simulink model "NOLCOlab2Q2"  (R2016b)
settings: Solver=ode4  StartTime=0.0  StopTime=10.0  FixedStep=0.001  RelTol=1e-3
settings Model: Creator=akshita_jain  LastModifiedBy=akshita_jain

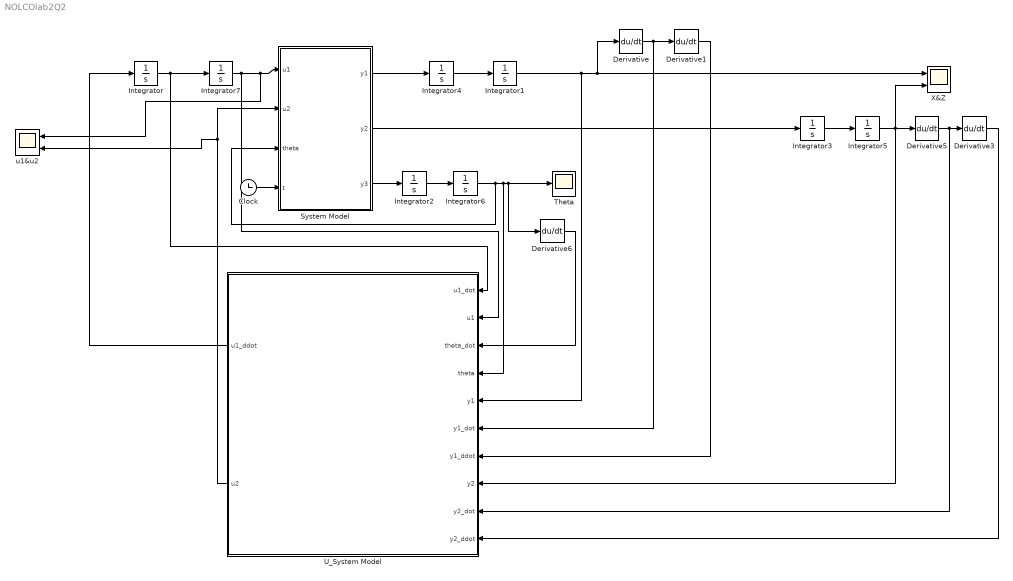
== system NOLCOlab2Q2 ==
  Clock : Clock
  Derivative{,1,3,5..6} (5 alike) : Derivative
  Integrator{,2..3,5..6} (5 alike) : Integrator
  Integrator1 : Integrator  InitialCondition=1
  Integrator4 : Integrator  InitialCondition=1
  Integrator7 : Integrator  InitialCondition=1
  System Model : MATLAB Function  TreatAsAtomicUnit=on
  Theta : Scope
  U_System Model : MATLAB Function  TreatAsAtomicUnit=on
  X&Z : Scope  NumInputPorts=2
  u1&u2 : Scope  NumInputPorts=2
  wires:
  System Model/2(y2) -> Integrator3/1
  System Model/3(y3) -> Integrator2/1
  U_System Model/1(u1_ddot) -> Integrator/1
  Integrator1/1 -> X&Z/1, Derivative/1, U_System Model/5(y1)
  Integrator2/1 -> Integrator6/1
  Integrator/1 -> U_System Model/1(u1_dot), Integrator7/1
  Integrator7/1 -> U_System Model/2(u1), u1&u2/1, System Model/1(u1)
  System Model/1(y1) -> Integrator4/1
  Integrator4/1 -> Integrator1/1
  Derivative/1 -> U_System Model/6(y1_dot), Derivative1/1
  Derivative1/1 -> U_System Model/7(y1_ddot)
  Integrator3/1 -> Integrator5/1
  Integrator5/1 -> X&Z/2, Derivative5/1, U_System Model/8(y2)
  Derivative5/1 -> U_System Model/9(y2_dot), Derivative3/1
  Derivative3/1 -> U_System Model/10(y2_ddot)
  U_System Model/2(u2) -> u1&u2/2, System Model/2(u2)
  Derivative6/1 -> U_System Model/3(theta_dot)
  Integrator6/1 -> System Model/3(theta), U_System Model/4(theta), Derivative6/1, Theta/1
  Clock/1 -> System Model/4(t)

== matlab function NOLCOlab2Q2/U_System Model ==
  data: u1_dot input; u1 input; theta_dot input; u1_ddot output; theta input; u2 output; y1 input; y1_dot input; y1_ddot input; y2 input; y2_dot input; y2_ddot input
function [u1_ddot,u2]= fcn(u1_dot,u1,theta_dot,theta,y1,y1_dot,y1_ddot,y2,y2_dot,y2_ddot)
% Gain Values:
k1 = 4;
k2 = 6;
k3 = 4;
k4 = 1;
% y_dddot calculations(differential equations)
y1_dddot = -u1_dot*sin(theta) - u1*theta_dot*cos(theta);
y2_dddot = u1_dot*cos(theta) - u1*theta_dot*sin(theta);

% Alpha Matrix
alpha = [-2*u1_dot*cos(theta)*theta_dot + u1*sin(theta)*(theta_dot^2);
        -2*u1_dot*sin(theta)*theta_dot - u1*cos(theta)*(theta_dot^2)];
% Beta Matrix
beta = [-sin(theta) -u1*cos(theta); cos(theta) -u1*sin(theta)];

% Gain(Output) Matrix
gain = [-k1*y1_dddot - k2*y1_ddot - k3*y1_dot - k4*y1; -k1*y2_dddot - k2*y2_ddot - k3*y2_dot - k4*y2];

u = beta^-1 * (-alpha+gain);
u1_ddot = u(1);
u2 = u(2);
end

== matlab function NOLCOlab2Q2/System Model ==
  data: u1 input; y1 output; u2 input; theta input; y2 output; y3 output; t input
function [y1,y2,y3]= fcn(u1,u2,theta,t)
del_t = 0;
x_ddot = -u1*sin(theta);
z_ddot = cos(theta)*u1 - 1;
theta_ddot = u2 + del_t*sin(t);
y1 = x_ddot;
y2 = z_ddot;
y3 = theta_ddot;
end
